simulink model "Cylinder_v1"  (R2023a)
settings: Solver=VariableStepAuto  StartTime=0.0  StopTime=10  RelTol=1e-3
values from neighbouring files (symbols this model uses):
  A_A = pi/4 * D^2    (= 0.000804247719319)    [system_parameters.m]
  A_B = A_A - pi/4 * d^2    (= 0.00049008845396)    [system_parameters.m]
  K_f = 1.6e9    (= 1600000000)    [system_parameters.m]
  m = 234    [system_parameters.m]
  omega = sqrt(k_tot / m)    [system_parameters.m]
  V_0_A = V_0_A_0 + V_pipe    (= 8.80230016469e-05)    [system_parameters.m]
  V_0_B = V_0_B_0 + V_pipe    (= 8.68230016469e-05)    [system_parameters.m]
  x_0 = 0.5    [system_parameters.m]
  x_max = 1.0    (= 1)    [system_parameters.m]
settings Model: Creator=porterf1  LastModifiedBy=porterf1

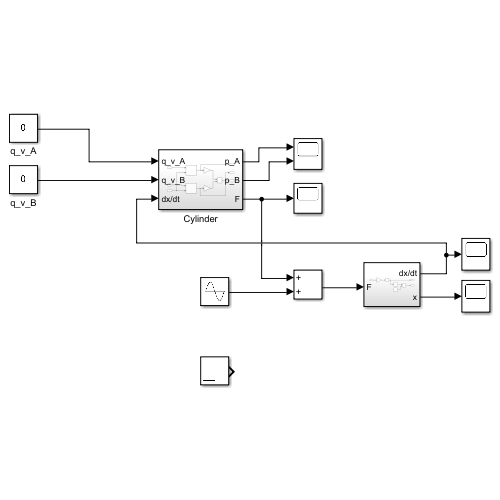
[thumbnail: Simulink's stored preview of the top-level diagram]
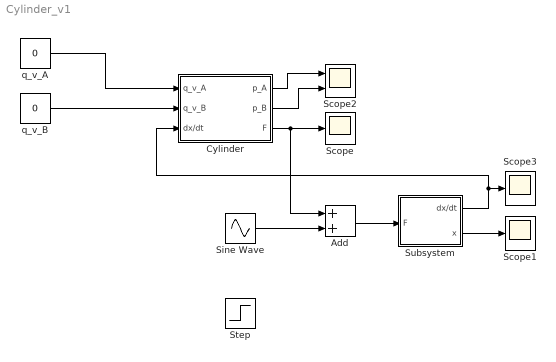
== system Cylinder_v1 ==
  Add : Sum
  Cylinder : Subsystem
  Scope : Scope
  Scope1 : Scope
  Scope2 : Scope  NumInputPorts=2
  Scope3 : Scope
  Sine Wave : Sin  Frequency=omega  SampleTime=0
  Step : Step  Time=0  After=100  SampleTime=0
  Subsystem : Subsystem
  q_v_A : Constant  Value=0
  q_v_B : Constant  Value=0
  wires:
  Cylinder/3(F) -> Add/1, Scope/1
  q_v_A/1 -> Cylinder/1(q_v_A)
  q_v_B/1 -> Cylinder/2(q_v_B)
  Subsystem/2(x) -> Scope1/1
  Cylinder/1(p_A) -> Scope2/1
  Cylinder/2(p_B) -> Scope2/2
  Add/1 -> Subsystem/1(F)
  Subsystem/1(dx/dt) -> Scope3/1, Cylinder/3(dx/dt)
  Sine Wave/1 -> Add/2

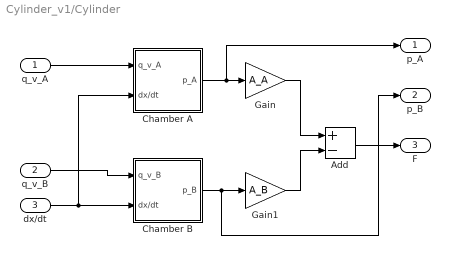
== system Cylinder_v1/Cylinder ==
  q_v_A : Inport
  q_v_B : Inport  Port=2
  dx/dt : Inport  Port=3
  Add : Sum  Inputs=+-
  Chamber A : Subsystem
  Chamber B : Subsystem
  Gain : Gain  Gain=A_A
  Gain1 : Gain  Gain=A_B
  p_A : Outport
  p_B : Outport  Port=2
  F : Outport  Port=3
  wires:
  Gain/1 -> Add/1
  Chamber B/1(p_B) -> p_B/1, Gain1/1
  Chamber A/1(p_A) -> p_A/1, Gain/1
  q_v_B/1 -> Chamber B/1(q_v_B)
  dx/dt/1 -> Chamber A/2(dx/dt), Chamber B/2(dx/dt)
  Add/1 -> F/1
  q_v_A/1 -> Chamber A/1(q_v_A)
  Gain1/1 -> Add/2

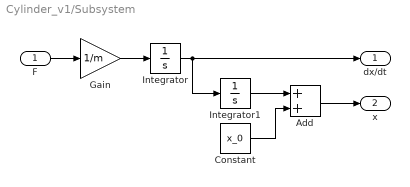
== system Cylinder_v1/Subsystem ==
  F : Inport
  Add : Sum
  Constant : Constant  Value=x_0
  Gain : Gain  Gain=1/m
  Integrator : Integrator
  Integrator1 : Integrator
  dx/dt : Outport
  x : Outport  Port=2
  wires:
  Integrator1/1 -> Add/1
  Constant/1 -> Add/2
  Add/1 -> x/1
  F/1 -> Gain/1
  Integrator/1 -> dx/dt/1, Integrator1/1
  Gain/1 -> Integrator/1

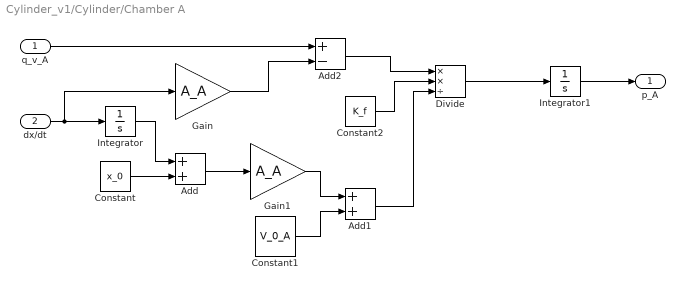
== system Cylinder_v1/Cylinder/Chamber A ==
  q_v_A : Inport
  dx/dt : Inport  Port=2
  Add : Sum
  Add1 : Sum
  Add2 : Sum  Inputs=+-
  Constant : Constant  Value=x_0
  Constant1 : Constant  Value=V_0_A
  Constant2 : Constant  Value=K_f
  Divide : Product  Inputs=**/
  Gain : Gain  Gain=A_A
  Gain1 : Gain  Gain=A_A
  Integrator : Integrator
  Integrator1 : Integrator
  p_A : Outport
  wires:
  dx/dt/1 -> Gain/1, Integrator/1
  Integrator/1 -> Add/1
  Constant/1 -> Add/2
  Add/1 -> Gain1/1
  Gain1/1 -> Add1/1
  Constant1/1 -> Add1/2
  Gain/1 -> Add2/2
  q_v_A/1 -> Add2/1
  Integrator1/1 -> p_A/1
  Add2/1 -> Divide/1
  Add1/1 -> Divide/3
  Divide/1 -> Integrator1/1
  Constant2/1 -> Divide/2

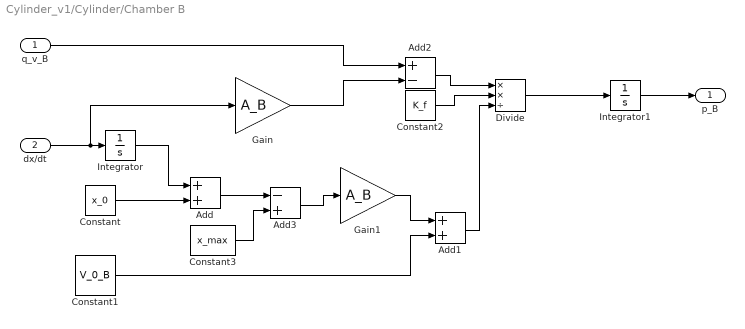
== system Cylinder_v1/Cylinder/Chamber B ==
  q_v_B : Inport
  dx/dt : Inport  Port=2
  Add : Sum
  Add1 : Sum
  Add2 : Sum  Inputs=+-
  Add3 : Sum  Inputs=-+
  Constant : Constant  Value=x_0
  Constant1 : Constant  Value=V_0_B
  Constant2 : Constant  Value=K_f
  Constant3 : Constant  Value=x_max
  Divide : Product  Inputs=**/
  Gain : Gain  Gain=A_B
  Gain1 : Gain  Gain=A_B
  Integrator : Integrator
  Integrator1 : Integrator
  p_B : Outport
  wires:
  dx/dt/1 -> Gain/1, Integrator/1
  Integrator/1 -> Add/1
  Constant/1 -> Add/2
  Gain1/1 -> Add1/1
  Constant1/1 -> Add1/2
  Gain/1 -> Add2/2
  q_v_B/1 -> Add2/1
  Integrator1/1 -> p_B/1
  Add2/1 -> Divide/1
  Add1/1 -> Divide/3
  Divide/1 -> Integrator1/1
  Constant2/1 -> Divide/2
  Add/1 -> Add3/1
  Add3/1 -> Gain1/1
  Constant3/1 -> Add3/2
